simulink model "lambda_threshold_diagnostic"  (R2025b)
settings: Solver=VariableStepAuto  StartTime=0.0  StopTime=300  RelTol=1e-3
libraries: simulink x2
settings Model: Creator=fedi  LastModifiedBy=fedi

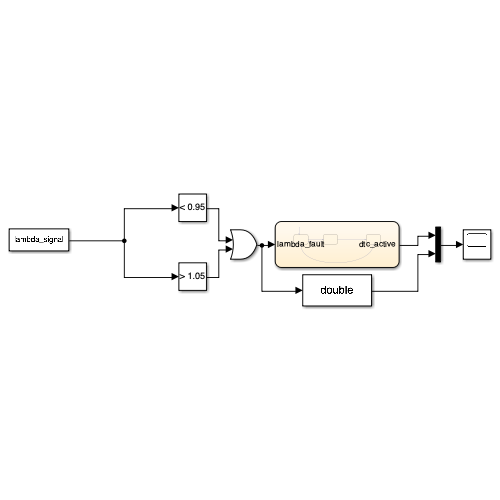
[thumbnail: Simulink's stored preview of the top-level diagram]
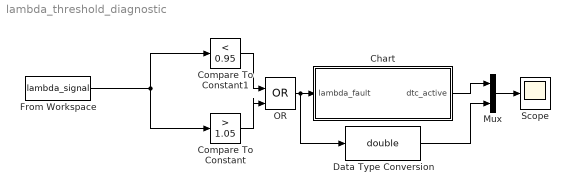
== system lambda_threshold_diagnostic ==
  Chart : Stateflow chart  TreatAsAtomicUnit=on
  Compare To Constant : simulink/Logic and Bit Operations/Compare To Constant  relop=>  const=1.05  OutDataTypeStr=boolean
  Compare To Constant1 : simulink/Logic and Bit Operations/Compare To Constant  relop=<  const=0.95  OutDataTypeStr=boolean
  Data Type Conversion : DataTypeConversion  OutDataTypeStr=double  SaturateOnIntegerOverflow=off  RndMeth=Floor
  From Workspace : FromWorkspace  VariableName=lambda_signal
  Mux : Mux  Inputs=2
  OR : Logic  Operator=OR  IconShape=distinctive  AllPortsSameDT=off  OutDataTypeStr=boolean
  Scope : Scope
      settings: ActiveDisplayYMinimum=-0.12499999999999997  ActiveDisplayYMaximum=1.125
  wires:
  From Workspace/1 -> Compare To Constant1/1, Compare To Constant/1
  Compare To Constant1/1 -> OR/1
  Compare To Constant/1 -> OR/2
  OR/1 -> Data Type Conversion/1, Chart/1(lambda_fault)
  Mux/1 -> Scope/1
  Chart/1(dtc_active) -> Mux/1
  Data Type Conversion/1 -> Mux/2

== stateflow chart lambda_threshold_diagnostic/Chart ==
  state NORMAL
    entry:
    dtc_active = 0;
  state PENDING
    entry:
    dtc_active = 0;
  state FAULT
    entry:
    dtc_active = 1;
  (default) -> NORMAL
  NORMAL -> PENDING : [lambda_fault]
  PENDING -> FAULT [order 1] : [lambda_fault && after(5, sec)]
  PENDING -> NORMAL [order 2] : [~lambda_fault]
  FAULT -> NORMAL : [~lambda_fault]
  data: lambda_fault input =boolean; dtc_active output
